simulink model "dcMotor_m"  (R2024a)
settings: Solver=VariableStepAuto  StartTime=0.0  StopTime=10.0  RelTol=1e-3
undefined symbols (not defined in the file): J, K_b, K_f, K_m, L, R
settings Model: Creator=Peter  LastModifiedBy=Peter

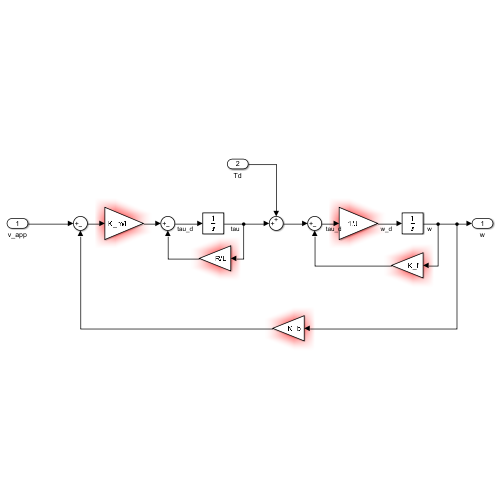
[thumbnail: Simulink's stored preview of the top-level diagram]
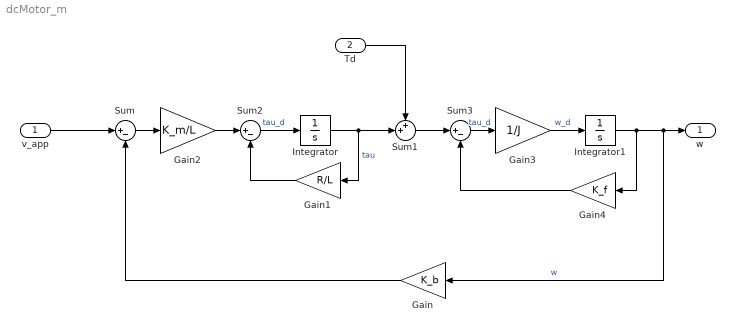
== system dcMotor_m ==
  v_app : Inport
  Td : Inport  Port=2
  Gain : Gain  Gain=K_b
  Gain1 : Gain  Gain=R/L
  Gain2 : Gain  Gain=K_m/L
  Gain3 : Gain  Gain=1/J
  Gain4 : Gain  Gain=K_f
  Integrator : Integrator
  Integrator1 : Integrator
  Sum : Sum  Inputs=|+-
  Sum1 : Sum  Inputs=++|
  Sum2 : Sum  Inputs=|+-
  Sum3 : Sum  Inputs=|+-
  w : Outport
  wires:
  v_app/1 -> Sum/1
  Gain/1 -> Sum/2
  Integrator/1 -> Sum1/2, Gain1/1  "tau"
  Sum2/1 -> Integrator/1  "tau_d"
  Sum/1 -> Gain2/1
  Gain2/1 -> Sum2/1
  Gain1/1 -> Sum2/2
  Td/1 -> Sum1/1
  Sum1/1 -> Sum3/1
  Integrator1/1 -> Gain/1, w/1, Gain4/1  "w"
  Gain3/1 -> Integrator1/1  "w_d"
  Gain4/1 -> Sum3/2
  Sum3/1 -> Gain3/1  "tau_d"
